simulink library "halout"  (R2021b)
settings: Solver=VariableStepAuto  StartTime=0.0  StopTime=10.0  RelTol=1e-3
undefined symbols (not defined in the file): C_TASK_5MS_S, FALSE, KHAL_CAN1FDAPS3E2E_flg, KHAL_CAN1FDAPS3TxReq_flg, KHAL_CAN1FDVCU2E2E_flg, KHAL_CAN1FDVCU2TxReq_flg, KHAL_CAN1FDVCU3E2E_flg, KHAL_CAN1FDVCU3TxReq_flg, KHAL_CAN1TxReq_flg, KHAL_CAN2TxReq_flg, KHAL_CAN3FDVCU1TxReq_flg, KHAL_CAN3FDVCU2E2E_flg, KHAL_CAN3FDVCU2TxReq_flg, KHAL_CAN3TxReq_flg, KHAL_CAN4FDVCU1E2E_flg, KHAL_CAN4FDVCU1TxReq_flg, KHAL_CAN4TxReq_flg, KHAL_CAN5TxReq_flg, ONE_INT, TRUE, ZERO_INT
libraries: FVT_lib x383, simulink x179
(part 14 of 20)

== system halout/HAL_OUT/CAN2/FD_BCM2_0x217/AmbLightBreath2 ==
  AmbLightBreath2 : Inport
  Data Type Conversion : DataTypeConversion  OutDataTypeStr=uint8  RndMeth=Round
  CAN2_AmbLightBreath2 : Outport
  wires:
  Data Type Conversion/1 -> CAN2_AmbLightBreath2/1
  AmbLightBreath2/1 -> Data Type Conversion/1

== system halout/HAL_OUT/CAN2/FD_BCM2_0x217/AmbLightBreath3 ==
  AmbLightBreath3 : Inport
  Data Type Conversion : DataTypeConversion  OutDataTypeStr=uint8  RndMeth=Round
  CAN2_AmbLightBreath3 : Outport
  wires:
  Data Type Conversion/1 -> CAN2_AmbLightBreath3/1
  AmbLightBreath3/1 -> Data Type Conversion/1

== system halout/HAL_OUT/CAN2/FD_BCM2_0x217/AmbLightBrightness1 ==
  AmbLightBrightness1 : Inport
  Data Type Conversion : DataTypeConversion  OutDataTypeStr=uint8  RndMeth=Round
  CAN2_AmbLightBrightness1 : Outport
  wires:
  Data Type Conversion/1 -> CAN2_AmbLightBrightness1/1
  AmbLightBrightness1/1 -> Data Type Conversion/1

== system halout/HAL_OUT/CAN2/FD_BCM2_0x217/AmbLightBrightness2 ==
  AmbLightBrightness2 : Inport
  Data Type Conversion : DataTypeConversion  OutDataTypeStr=uint8  RndMeth=Round
  CAN2_AmbLightBrightness2 : Outport
  wires:
  Data Type Conversion/1 -> CAN2_AmbLightBrightness2/1
  AmbLightBrightness2/1 -> Data Type Conversion/1

== system halout/HAL_OUT/CAN2/FD_BCM2_0x217/AmbLightBrightness3 ==
  AmbLightBrightness3 : Inport
  Data Type Conversion : DataTypeConversion  OutDataTypeStr=uint8  RndMeth=Round
  CAN2_AmbLightBrightness3 : Outport
  wires:
  Data Type Conversion/1 -> CAN2_AmbLightBrightness3/1
  AmbLightBrightness3/1 -> Data Type Conversion/1

== system halout/HAL_OUT/CAN2/FD_BCM2_0x217/AmbLightColor1 ==
  AmbLightColor1 : Inport
  Data Type Conversion : DataTypeConversion  OutDataTypeStr=uint8  RndMeth=Round
  CAN2_AmbLightColor1 : Outport
  wires:
  Data Type Conversion/1 -> CAN2_AmbLightColor1/1
  AmbLightColor1/1 -> Data Type Conversion/1

== system halout/HAL_OUT/CAN2/FD_BCM2_0x217/AmbLightColor2 ==
  AmbLightColor2 : Inport
  Data Type Conversion : DataTypeConversion  OutDataTypeStr=uint8  RndMeth=Round
  CAN2_AmbLightColor2 : Outport
  wires:
  Data Type Conversion/1 -> CAN2_AmbLightColor2/1
  AmbLightColor2/1 -> Data Type Conversion/1

== system halout/HAL_OUT/CAN2/FD_BCM2_0x217/AmbLightColor3 ==
  AmbLightColor3 : Inport
  Data Type Conversion : DataTypeConversion  OutDataTypeStr=uint8  RndMeth=Round
  CAN2_AmbLightColor3 : Outport
  wires:
  Data Type Conversion/1 -> CAN2_AmbLightColor3/1
  AmbLightColor3/1 -> Data Type Conversion/1

== system halout/HAL_OUT/CAN2/FD_BCM2_0x217/LampPwr ==
  LampPwr : Inport
  Data Type Conversion : DataTypeConversion  OutDataTypeStr=uint8  RndMeth=Round
  CAN2_LampPwr : Outport
  wires:
  Data Type Conversion/1 -> CAN2_LampPwr/1
  LampPwr/1 -> Data Type Conversion/1

== system halout/HAL_OUT/CAN2/FD_BCM2_0x217/User1AmbLightColor ==
  User1AmbLightColor : Inport
  Data Type Conversion : DataTypeConversion  OutDataTypeStr=uint8  RndMeth=Round
  CAN2_User1AmbLightColor : Outport
  wires:
  Data Type Conversion/1 -> CAN2_User1AmbLightColor/1
  User1AmbLightColor/1 -> Data Type Conversion/1

== system halout/HAL_OUT/CAN2/FD_BCM2_0x217/User1DrAmbLightBrightness ==
  User1DrAmbLightBrightness : Inport
  Data Type Conversion : DataTypeConversion  OutDataTypeStr=uint8  RndMeth=Round
  CAN2_User1DrAmbLightBrightness : Outport
  wires:
  Data Type Conversion/1 -> CAN2_User1DrAmbLightBrightness/1
  User1DrAmbLightBrightness/1 -> Data Type Conversion/1

== system halout/HAL_OUT/CAN2/FD_BCM2_0x217/User1IPAmbLightBrightness ==
  User1IPAmbLightBrightness : Inport
  Data Type Conversion : DataTypeConversion  OutDataTypeStr=uint8  RndMeth=Round
  CAN2_User1IPAmbLightBrightness : Outport
  wires:
  Data Type Conversion/1 -> CAN2_User1IPAmbLightBrightness/1
  User1IPAmbLightBrightness/1 -> Data Type Conversion/1

== system halout/HAL_OUT/CAN2/FD_BCM2_0x217/User2AmbLightColor ==
  User2AmbLightColor : Inport
  Data Type Conversion : DataTypeConversion  OutDataTypeStr=uint8  RndMeth=Round
  CAN2_User2AmbLightColor : Outport
  wires:
  Data Type Conversion/1 -> CAN2_User2AmbLightColor/1
  User2AmbLightColor/1 -> Data Type Conversion/1

== system halout/HAL_OUT/CAN2/FD_BCM2_0x217/User2DrAmbLightBrightness ==
  User2DrAmbLightBrightness : Inport
  Data Type Conversion : DataTypeConversion  OutDataTypeStr=uint8  RndMeth=Round
  CAN2_User2DrAmbLightBrightness : Outport
  wires:
  Data Type Conversion/1 -> CAN2_User2DrAmbLightBrightness/1
  User2DrAmbLightBrightness/1 -> Data Type Conversion/1

== system halout/HAL_OUT/CAN2/FD_BCM2_0x217/User2IPAmbLightBrightness ==
  User2IPAmbLightBrightness : Inport
  Data Type Conversion : DataTypeConversion  OutDataTypeStr=uint8  RndMeth=Round
  CAN2_User2IPAmbLightBrightness : Outport
  wires:
  Data Type Conversion/1 -> CAN2_User2IPAmbLightBrightness/1
  User2IPAmbLightBrightness/1 -> Data Type Conversion/1

== system halout/HAL_OUT/CAN2/FD_BCM2_0x217/User3AmbLightColor ==
  User3AmbLightColor : Inport
  Data Type Conversion : DataTypeConversion  OutDataTypeStr=uint8  RndMeth=Round
  CAN2_User3AmbLightColor : Outport
  wires:
  Data Type Conversion/1 -> CAN2_User3AmbLightColor/1
  User3AmbLightColor/1 -> Data Type Conversion/1

== system halout/HAL_OUT/CAN2/FD_BCM2_0x217/User3DrAmbLightBrightness ==
  User3DrAmbLightBrightness : Inport
  Data Type Conversion : DataTypeConversion  OutDataTypeStr=uint8  RndMeth=Round
  CAN2_User3DrAmbLightBrightness : Outport
  wires:
  Data Type Conversion/1 -> CAN2_User3DrAmbLightBrightness/1
  User3DrAmbLightBrightness/1 -> Data Type Conversion/1

== system halout/HAL_OUT/CAN2/FD_BCM2_0x217/User3IPAmbLightBrightness ==
  User3IPAmbLightBrightness : Inport
  Data Type Conversion : DataTypeConversion  OutDataTypeStr=uint8  RndMeth=Round
  CAN2_User3IPAmbLightBrightness : Outport
  wires:
  Data Type Conversion/1 -> CAN2_User3IPAmbLightBrightness/1
  User3IPAmbLightBrightness/1 -> Data Type Conversion/1

== system halout/HAL_OUT/CAN2/FD_BCM2_0x217/User4AmbLightColor ==
  User4AmbLightColor : Inport
  Data Type Conversion : DataTypeConversion  OutDataTypeStr=uint8  RndMeth=Round
  CAN2_User4AmbLightColor : Outport
  wires:
  Data Type Conversion/1 -> CAN2_User4AmbLightColor/1
  User4AmbLightColor/1 -> Data Type Conversion/1

== system halout/HAL_OUT/CAN2/FD_BCM2_0x217/User4DrAmbLightBrightness ==
  User4DrAmbLightBrightness : Inport
  Data Type Conversion : DataTypeConversion  OutDataTypeStr=uint8  RndMeth=Round
  CAN2_User4DrAmbLightBrightness : Outport
  wires:
  Data Type Conversion/1 -> CAN2_User4DrAmbLightBrightness/1
  User4DrAmbLightBrightness/1 -> Data Type Conversion/1

== system halout/HAL_OUT/CAN2/FD_BCM2_0x217/User4IPAmbLightBrightness ==
  User4IPAmbLightBrightness : Inport
  Data Type Conversion : DataTypeConversion  OutDataTypeStr=uint8  RndMeth=Round
  CAN2_User4IPAmbLightBrightness : Outport
  wires:
  Data Type Conversion/1 -> CAN2_User4IPAmbLightBrightness/1
  User4IPAmbLightBrightness/1 -> Data Type Conversion/1

== system halout/HAL_OUT/CAN2/FD_BCM2_0x217/User5AmbLightColor ==
  User5AmbLightColor : Inport
  Data Type Conversion : DataTypeConversion  OutDataTypeStr=uint8  RndMeth=Round
  CAN2_User5AmbLightColor : Outport
  wires:
  Data Type Conversion/1 -> CAN2_User5AmbLightColor/1
  User5AmbLightColor/1 -> Data Type Conversion/1

== system halout/HAL_OUT/CAN2/FD_BCM2_0x217/User5DrAmbLightBrightness ==
  User5DrAmbLightBrightness : Inport
  Data Type Conversion : DataTypeConversion  OutDataTypeStr=uint8  RndMeth=Round
  CAN2_User5DrAmbLightBrightness : Outport
  wires:
  Data Type Conversion/1 -> CAN2_User5DrAmbLightBrightness/1
  User5DrAmbLightBrightness/1 -> Data Type Conversion/1

== system halout/HAL_OUT/CAN2/FD_BCM2_0x217/User5IPAmbLightBrightness ==
  User5IPAmbLightBrightness : Inport
  Data Type Conversion : DataTypeConversion  OutDataTypeStr=uint8  RndMeth=Round
  CAN2_User5IPAmbLightBrightness : Outport
  wires:
  Data Type Conversion/1 -> CAN2_User5IPAmbLightBrightness/1
  User5IPAmbLightBrightness/1 -> Data Type Conversion/1

== system halout/HAL_OUT/CAN2/FD_BCM2_0x217/User6AmbLightColor ==
  User6AmbLightColor : Inport
  Data Type Conversion : DataTypeConversion  OutDataTypeStr=uint8  RndMeth=Round
  CAN2_User6AmbLightColor : Outport
  wires:
  Data Type Conversion/1 -> CAN2_User6AmbLightColor/1
  User6AmbLightColor/1 -> Data Type Conversion/1

== system halout/HAL_OUT/CAN2/FD_BCM2_0x217/User6DrAmbLightBrightness ==
  User6DrAmbLightBrightness : Inport
  Data Type Conversion : DataTypeConversion  OutDataTypeStr=uint8  RndMeth=Round
  CAN2_User6DrAmbLightBrightness : Outport
  wires:
  Data Type Conversion/1 -> CAN2_User6DrAmbLightBrightness/1
  User6DrAmbLightBrightness/1 -> Data Type Conversion/1

== system halout/HAL_OUT/CAN2/FD_BCM2_0x217/User6IPAmbLightBrightness ==
  User6IPAmbLightBrightness : Inport
  Data Type Conversion : DataTypeConversion  OutDataTypeStr=uint8  RndMeth=Round
  CAN2_User6IPAmbLightBrightness : Outport
  wires:
  Data Type Conversion/1 -> CAN2_User6IPAmbLightBrightness/1
  User6IPAmbLightBrightness/1 -> Data Type Conversion/1

== system halout/HAL_OUT/CAN2/FD_THCM1_0x182/BatteryMode ==
  BatteryMode : Inport
  Data Type Conversion : DataTypeConversion  OutDataTypeStr=uint8  RndMeth=Round
  CAN2_BatteryMode : Outport
  wires:
  Data Type Conversion/1 -> CAN2_BatteryMode/1
  BatteryMode/1 -> Data Type Conversion/1

== system halout/HAL_OUT/CAN2/FD_THCM1_0x182/CCUACLampSts ==
  CCUACLampSts : Inport
  Data Type Conversion : DataTypeConversion  OutDataTypeStr=uint8  RndMeth=Round
  CAN2_CCU_ACLampSts : Outport
  wires:
  Data Type Conversion/1 -> CAN2_CCU_ACLampSts/1
  CCUACLampSts/1 -> Data Type Conversion/1

== system halout/HAL_OUT/CAN2/FD_THCM1_0x182/CCUACMaxLampSts ==
  CCUACMaxLampSts : Inport
  Data Type Conversion : DataTypeConversion  OutDataTypeStr=uint8  RndMeth=Round
  CAN2_CCU_ACMaxLampSts : Outport
  wires:
  Data Type Conversion/1 -> CAN2_CCU_ACMaxLampSts/1
  CCUACMaxLampSts/1 -> Data Type Conversion/1

== system halout/HAL_OUT/CAN2/FD_THCM1_0x182/CCUAutoLampSts ==
  CCUAutoLampSts : Inport
  Data Type Conversion : DataTypeConversion  OutDataTypeStr=uint8  RndMeth=Round
  CAN2_CCU_AutoLampSts : Outport
  wires:
  Data Type Conversion/1 -> CAN2_CCU_AutoLampSts/1
  CCUAutoLampSts/1 -> Data Type Conversion/1

== system halout/HAL_OUT/CAN2/FD_THCM1_0x182/CCUAutoMidLampSts ==
  CCUAutoMidLampSts : Inport
  Data Type Conversion : DataTypeConversion  OutDataTypeStr=uint8  RndMeth=Round
  CAN2_CCU_AutoMidLampSts : Outport
  wires:
  Data Type Conversion/1 -> CAN2_CCU_AutoMidLampSts/1
  CCUAutoMidLampSts/1 -> Data Type Conversion/1

== system halout/HAL_OUT/CAN2/FD_THCM1_0x182/CCUDispalyRequest ==
  CCUDispalyRequest : Inport
  Data Type Conversion : DataTypeConversion  OutDataTypeStr=uint8  RndMeth=Round
  CAN2_CCU_Dispaly_Request : Outport
  wires:
  Data Type Conversion/1 -> CAN2_CCU_Dispaly_Request/1
  CCUDispalyRequest/1 -> Data Type Conversion/1

== system halout/HAL_OUT/CAN2/FD_THCM1_0x182/CCUEcoSts ==
  CCUEcoSts : Inport
  Data Type Conversion : DataTypeConversion  OutDataTypeStr=uint8  RndMeth=Round
  CAN2_CCU_EcoSts : Outport
  wires:
  Data Type Conversion/1 -> CAN2_CCU_EcoSts/1
  CCUEcoSts/1 -> Data Type Conversion/1

== system halout/HAL_OUT/CAN2/FD_THCM1_0x182/CCUFrtOnOffLampSts ==
  CCUFrtOnOffLampSts : Inport
  Data Type Conversion : DataTypeConversion  OutDataTypeStr=uint8  RndMeth=Round
  CAN2_CCU_FrtOnOffLampSts : Outport
  wires:
  Data Type Conversion/1 -> CAN2_CCU_FrtOnOffLampSts/1
  CCUFrtOnOffLampSts/1 -> Data Type Conversion/1

== system halout/HAL_OUT/CAN2/FD_THCM1_0x182/CCUHEATMaxLampSts ==
  CCUHEATMaxLampSts : Inport
  Data Type Conversion : DataTypeConversion  OutDataTypeStr=uint8  RndMeth=Round
  CAN2_CCU_HEATMaxLampSts : Outport
  wires:
  Data Type Conversion/1 -> CAN2_CCU_HEATMaxLampSts/1
  CCUHEATMaxLampSts/1 -> Data Type Conversion/1

== system halout/HAL_OUT/CAN2/FD_THCM1_0x182/CCURrOnOffLampSts ==
  CCURrOnOffLampSts : Inport
  Data Type Conversion : DataTypeConversion  OutDataTypeStr=uint8  RndMeth=Round
  CAN2_CCU_RrOnOffLampSts : Outport
  wires:
  Data Type Conversion/1 -> CAN2_CCU_RrOnOffLampSts/1
  CCURrOnOffLampSts/1 -> Data Type Conversion/1

== system halout/HAL_OUT/CAN2/FD_THCM1_0x182/CCUSyncLampSts ==
  CCUSyncLampSts : Inport
  Data Type Conversion : DataTypeConversion  OutDataTypeStr=uint8  RndMeth=Round
  CAN2_CCU_SyncLampSts : Outport
  wires:
  Data Type Conversion/1 -> CAN2_CCU_SyncLampSts/1
  CCUSyncLampSts/1 -> Data Type Conversion/1

== system halout/HAL_OUT/CAN2/FD_THCM1_0x182/CabinMode ==
  CabinMode : Inport
  Data Type Conversion : DataTypeConversion  OutDataTypeStr=uint8  RndMeth=Round
  CAN2_CabinMode : Outport
  wires:
  Data Type Conversion/1 -> CAN2_CabinMode/1
  CabinMode/1 -> Data Type Conversion/1

== system halout/HAL_OUT/CAN2/FD_THCM1_0x182/EDriveMode ==
  EDriveMode : Inport
  Data Type Conversion : DataTypeConversion  OutDataTypeStr=uint8  RndMeth=Round
  CAN2_EDriveMode : Outport
  wires:
  Data Type Conversion/1 -> CAN2_EDriveMode/1
  EDriveMode/1 -> Data Type Conversion/1

== system halout/HAL_OUT/CAN2/FD_THCM1_0x182/FDAGSCmd ==
  FDAGSCmd : Inport
  Data Type Conversion : DataTypeConversion  OutDataTypeStr=uint8  RndMeth=Round
  CAN2_FD_AGS_Cmd : Outport
  wires:
  Data Type Conversion/1 -> CAN2_FD_AGS_Cmd/1
  FDAGSCmd/1 -> Data Type Conversion/1

== system halout/HAL_OUT/CAN2/FD_THCM1_0x182/FDRecyAutoCmd ==
  FDRecyAutoCmd : Inport
  Data Type Conversion : DataTypeConversion  OutDataTypeStr=uint8  RndMeth=Round
  CAN2_FD_RecyAuto_Cmd : Outport
  wires:
  Data Type Conversion/1 -> CAN2_FD_RecyAuto_Cmd/1
  FDRecyAutoCmd/1 -> Data Type Conversion/1

== system halout/HAL_OUT/CAN2/FD_THCM1_0x182/FrCoolantflow ==
  FrCoolantflow : Inport
  Data Type Conversion : DataTypeConversion  OutDataTypeStr=uint8  RndMeth=Round
  convert_out : FVT_lib/hal/convert_out  gain=0.25  offset=0
  CAN2_Fr_Coolantflow : Outport
  wires:
  Data Type Conversion/1 -> CAN2_Fr_Coolantflow/1
  convert_out/1 -> Data Type Conversion/1
  FrCoolantflow/1 -> convert_out/1

== system halout/HAL_OUT/CAN2/FD_THCM1_0x182/FrCoolanttemp ==
  FrCoolanttemp : Inport
  Data Type Conversion : DataTypeConversion  OutDataTypeStr=uint16  RndMeth=Round
  convert_out : FVT_lib/hal/convert_out  gain=1  offset=-40
  CAN2_Fr_Coolanttemp : Outport
  wires:
  Data Type Conversion/1 -> CAN2_Fr_Coolanttemp/1
  convert_out/1 -> Data Type Conversion/1
  FrCoolanttemp/1 -> convert_out/1

== system halout/HAL_OUT/CAN2/FD_THCM1_0x182/HPThermalRecoveryReq ==
  HPThermalRecoveryReq : Inport
  Data Type Conversion : DataTypeConversion  OutDataTypeStr=uint8  RndMeth=Round
  CAN2_HPThermalRecoveryReq : Outport
  wires:
  Data Type Conversion/1 -> CAN2_HPThermalRecoveryReq/1
  HPThermalRecoveryReq/1 -> Data Type Conversion/1

== system halout/HAL_OUT/CAN2/FD_THCM1_0x182/RrCoolantflow ==
  RrCoolantflow : Inport
  Data Type Conversion : DataTypeConversion  OutDataTypeStr=uint8  RndMeth=Round
  convert_out : FVT_lib/hal/convert_out  gain=0.25  offset=0
  CAN2_Rr_Coolantflow : Outport
  wires:
  Data Type Conversion/1 -> CAN2_Rr_Coolantflow/1
  convert_out/1 -> Data Type Conversion/1
  RrCoolantflow/1 -> convert_out/1

== system halout/HAL_OUT/CAN2/FD_THCM1_0x182/RrCoolanttemp ==
  RrCoolanttemp : Inport
  Data Type Conversion : DataTypeConversion  OutDataTypeStr=uint16  RndMeth=Round
  convert_out : FVT_lib/hal/convert_out  gain=1  offset=-40
  CAN2_Rr_Coolanttemp : Outport
  wires:
  Data Type Conversion/1 -> CAN2_Rr_Coolanttemp/1
  convert_out/1 -> Data Type Conversion/1
  RrCoolanttemp/1 -> convert_out/1

== system halout/HAL_OUT/CAN2/FD_THCM1_0x182/sigAirIntenZon1St ==
  sigAirIntenZon1St : Inport
  Data Type Conversion : DataTypeConversion  OutDataTypeStr=uint8  RndMeth=Round
  CAN2_sigAirIntenZon1St : Outport
  wires:
  Data Type Conversion/1 -> CAN2_sigAirIntenZon1St/1
  sigAirIntenZon1St/1 -> Data Type Conversion/1

== system halout/HAL_OUT/CAN2/FD_THCM1_0x182/sigAirIntenZon3St ==
  sigAirIntenZon3St : Inport
  Data Type Conversion : DataTypeConversion  OutDataTypeStr=uint8  RndMeth=Round
  CAN2_sigAirIntenZon3St : Outport
  wires:
  Data Type Conversion/1 -> CAN2_sigAirIntenZon3St/1
  sigAirIntenZon3St/1 -> Data Type Conversion/1

== system halout/HAL_OUT/CAN2/FD_THCM1_0x182/sigAmbAirT ==
  sigAmbAirT : Inport
  Data Type Conversion : DataTypeConversion  OutDataTypeStr=uint8  RndMeth=Round
  convert_out : FVT_lib/hal/convert_out  gain=0.5  offset=-40
  CAN2_sigAmbAirT : Outport
  wires:
  Data Type Conversion/1 -> CAN2_sigAmbAirT/1
  convert_out/1 -> Data Type Conversion/1
  sigAmbAirT/1 -> convert_out/1

== system halout/HAL_OUT/CAN2/FD_THCM1_0x182/sigCbnAirT ==
  sigCbnAirT : Inport
  Data Type Conversion : DataTypeConversion  OutDataTypeStr=uint8  RndMeth=Round
  convert_out : FVT_lib/hal/convert_out  gain=0.5  offset=-40
  CAN2_sigCbnAirT : Outport
  wires:
  Data Type Conversion/1 -> CAN2_sigCbnAirT/1
  convert_out/1 -> Data Type Conversion/1
  sigCbnAirT/1 -> convert_out/1

== system halout/HAL_OUT/CAN2/FD_THCM1_0x182/sigCbnPTCPwrAct ==
  sigCbnPTCPwrAct : Inport
  Data Type Conversion : DataTypeConversion  OutDataTypeStr=uint8  RndMeth=Round
  convert_out : FVT_lib/hal/convert_out  gain=50  offset=0
  CAN2_sigCbnPTCPwrAct : Outport
  wires:
  Data Type Conversion/1 -> CAN2_sigCbnPTCPwrAct/1
  convert_out/1 -> Data Type Conversion/1
  sigCbnPTCPwrAct/1 -> convert_out/1

== system halout/HAL_OUT/CAN2/FD_THCM1_0x182/sigCbnSolarLeft ==
  sigCbnSolarLeft : Inport
  Data Type Conversion : DataTypeConversion  OutDataTypeStr=uint8  RndMeth=Round
  convert_out : FVT_lib/hal/convert_out  gain=5  offset=0
  CAN2_sigCbnSolarLeft : Outport
  wires:
  Data Type Conversion/1 -> CAN2_sigCbnSolarLeft/1
  convert_out/1 -> Data Type Conversion/1
  sigCbnSolarLeft/1 -> convert_out/1

== system halout/HAL_OUT/CAN2/FD_THCM1_0x182/sigCbnSolarRight ==
  sigCbnSolarRight : Inport
  Data Type Conversion : DataTypeConversion  OutDataTypeStr=uint8  RndMeth=Round
  convert_out : FVT_lib/hal/convert_out  gain=5  offset=0
  CAN2_sigCbnSolarRight : Outport
  wires:
  Data Type Conversion/1 -> CAN2_sigCbnSolarRight/1
  convert_out/1 -> Data Type Conversion/1
  sigCbnSolarRight/1 -> convert_out/1

== system halout/HAL_OUT/CAN2/FD_THCM1_0x182/sigClmtCmprPwrAct ==
  sigClmtCmprPwrAct : Inport
  Data Type Conversion : DataTypeConversion  OutDataTypeStr=uint8  RndMeth=Round
  convert_out : FVT_lib/hal/convert_out  gain=50  offset=0
  CAN2_sigClmtCmprPwrAct : Outport
  wires:
  Data Type Conversion/1 -> CAN2_sigClmtCmprPwrAct/1
  convert_out/1 -> Data Type Conversion/1
  sigClmtCmprPwrAct/1 -> convert_out/1

== system halout/HAL_OUT/CAN2/FD_THCM1_0x182/sigClntTHvBattOut ==
  sigClntTHvBattOut : Inport
  Data Type Conversion : DataTypeConversion  OutDataTypeStr=uint8  RndMeth=Round
  convert_out : FVT_lib/hal/convert_out  gain=0.5  offset=-40
  CAN2_sigClntTHvBattOut : Outport
  wires:
  Data Type Conversion/1 -> CAN2_sigClntTHvBattOut/1
  convert_out/1 -> Data Type Conversion/1
  sigClntTHvBattOut/1 -> convert_out/1

== system halout/HAL_OUT/CAN2/FD_THCM1_0x182/sigDfrstSt ==
  sigDfrstSt : Inport
  Data Type Conversion : DataTypeConversion  OutDataTypeStr=uint8  RndMeth=Round
  CAN2_sigDfrstSt : Outport
  wires:
  Data Type Conversion/1 -> CAN2_sigDfrstSt/1
  sigDfrstSt/1 -> Data Type Conversion/1

== system halout/HAL_OUT/CAN2/FD_THCM1_0x182/sigHvacSt ==
  sigHvacSt : Inport
  Data Type Conversion : DataTypeConversion  OutDataTypeStr=uint8  RndMeth=Round
  CAN2_sigHvacSt : Outport
  wires:
  Data Type Conversion/1 -> CAN2_sigHvacSt/1
  sigHvacSt/1 -> Data Type Conversion/1

== system halout/HAL_OUT/CAN2/FD_THCM1_0x182/sigRecircSt ==
  sigRecircSt : Inport
  Data Type Conversion : DataTypeConversion  OutDataTypeStr=uint8  RndMeth=Round
  CAN2_sigRecircSt : Outport
  wires:
  Data Type Conversion/1 -> CAN2_sigRecircSt/1
  sigRecircSt/1 -> Data Type Conversion/1

== system halout/HAL_OUT/CAN2/FD_THCM1_0x182/sigSetTempZon1St ==
  sigSetTempZon1St : Inport
  Data Type Conversion : DataTypeConversion  OutDataTypeStr=uint8  RndMeth=Round
  convert_out : FVT_lib/hal/convert_out  gain=0.5  offset=17
  CAN2_sigSetTempZon1St : Outport
  wires:
  Data Type Conversion/1 -> CAN2_sigSetTempZon1St/1
  convert_out/1 -> Data Type Conversion/1
  sigSetTempZon1St/1 -> convert_out/1

== system halout/HAL_OUT/CAN2/FD_THCM1_0x182/sigSetTempZon2St ==
  sigSetTempZon2St : Inport
  Data Type Conversion : DataTypeConversion  OutDataTypeStr=uint8  RndMeth=Round
  convert_out : FVT_lib/hal/convert_out  gain=0.5  offset=17
  CAN2_sigSetTempZon2St : Outport
  wires:
  Data Type Conversion/1 -> CAN2_sigSetTempZon2St/1
  convert_out/1 -> Data Type Conversion/1
  sigSetTempZon2St/1 -> convert_out/1

== system halout/HAL_OUT/CAN2/FD_THCM1_0x182/sigSetTempZon3St ==
  sigSetTempZon3St : Inport
  Data Type Conversion : DataTypeConversion  OutDataTypeStr=uint8  RndMeth=Round
  convert_out : FVT_lib/hal/convert_out  gain=0.5  offset=17
  CAN2_sigSetTempZon3St : Outport
  wires:
  Data Type Conversion/1 -> CAN2_sigSetTempZon3St/1
  convert_out/1 -> Data Type Conversion/1
  sigSetTempZon3St/1 -> convert_out/1

== system halout/HAL_OUT/CAN2/FD_THCM1_0x182/sigWindDirZon1St ==
  sigWindDirZon1St : Inport
  Data Type Conversion : DataTypeConversion  OutDataTypeStr=uint8  RndMeth=Round
  CAN2_sigWindDirZon1St : Outport
  wires:
  Data Type Conversion/1 -> CAN2_sigWindDirZon1St/1
  sigWindDirZon1St/1 -> Data Type Conversion/1

== system halout/HAL_OUT/CAN2/FD_THCM1_0x182/sigWindDirZon3St ==
  sigWindDirZon3St : Inport
  Data Type Conversion : DataTypeConversion  OutDataTypeStr=uint8  RndMeth=Round
  CAN2_sigWindDirZon3St : Outport
  wires:
  Data Type Conversion/1 -> CAN2_sigWindDirZon3St/1
  sigWindDirZon3St/1 -> Data Type Conversion/1

== system halout/HAL_OUT/CAN2/FD_TPMS1_0x435/AutoLTips ==
  AutoLTips : Inport
  Data Type Conversion : DataTypeConversion  OutDataTypeStr=uint8  RndMeth=Round
  CAN2_AutoLTips : Outport
  wires:
  Data Type Conversion/1 -> CAN2_AutoLTips/1
  AutoLTips/1 -> Data Type Conversion/1

== system halout/HAL_OUT/CAN2/FD_TPMS1_0x435/CWheelTips ==
  CWheelTips : Inport
  Data Type Conversion : DataTypeConversion  OutDataTypeStr=uint8  RndMeth=Round
  CAN2_CWheelTips : Outport
  wires:
  Data Type Conversion/1 -> CAN2_CWheelTips/1
  CWheelTips/1 -> Data Type Conversion/1

== system halout/HAL_OUT/CAN2/FD_TPMS1_0x435/LFBatWarn ==
  LFBatWarn : Inport
  Data Type Conversion : DataTypeConversion  OutDataTypeStr=uint8  RndMeth=Round
  CAN2_LFBatWarn : Outport
  wires:
  Data Type Conversion/1 -> CAN2_LFBatWarn/1
  LFBatWarn/1 -> Data Type Conversion/1

== system halout/HAL_OUT/CAN2/FD_TPMS1_0x435/LFPressIndi ==
  LFPressIndi : Inport
  Data Type Conversion : DataTypeConversion  OutDataTypeStr=uint8  RndMeth=Round
  CAN2_LFPressIndi : Outport
  wires:
  Data Type Conversion/1 -> CAN2_LFPressIndi/1
  LFPressIndi/1 -> Data Type Conversion/1

== system halout/HAL_OUT/CAN2/FD_TPMS1_0x435/LFSensorFail ==
  LFSensorFail : Inport
  Data Type Conversion : DataTypeConversion  OutDataTypeStr=uint8  RndMeth=Round
  CAN2_LFSensorFail : Outport
  wires:
  Data Type Conversion/1 -> CAN2_LFSensorFail/1
  LFSensorFail/1 -> Data Type Conversion/1

== system halout/HAL_OUT/CAN2/FD_TPMS1_0x435/LFSensorMode ==
  LFSensorMode : Inport
  Data Type Conversion : DataTypeConversion  OutDataTypeStr=uint8  RndMeth=Round
  CAN2_LFSensorMode : Outport
  wires:
  Data Type Conversion/1 -> CAN2_LFSensorMode/1
  LFSensorMode/1 -> Data Type Conversion/1

== system halout/HAL_OUT/CAN2/FD_TPMS1_0x435/LFWheelDebug ==
  LFWheelDebug : Inport
  Data Type Conversion : DataTypeConversion  OutDataTypeStr=uint8  RndMeth=Round
  CAN2_LFWheelDebug : Outport
  wires:
  Data Type Conversion/1 -> CAN2_LFWheelDebug/1
  LFWheelDebug/1 -> Data Type Conversion/1

== system halout/HAL_OUT/CAN2/FD_TPMS1_0x435/LFWheelPSW ==
  LFWheelPSW : Inport
  Data Type Conversion : DataTypeConversion  OutDataTypeStr=uint8  RndMeth=Round
  CAN2_LFWheelPSW : Outport
  wires:
  Data Type Conversion/1 -> CAN2_LFWheelPSW/1
  LFWheelPSW/1 -> Data Type Conversion/1

== system halout/HAL_OUT/CAN2/FD_TPMS1_0x435/LFWheelPress ==
  LFWheelPress : Inport
  Data Type Conversion : DataTypeConversion  OutDataTypeStr=uint8  RndMeth=Round
  CAN2_LFWheelPress : Outport
  wires:
  Data Type Conversion/1 -> CAN2_LFWheelPress/1
  LFWheelPress/1 -> Data Type Conversion/1

== system halout/HAL_OUT/CAN2/FD_TPMS1_0x435/LFWheelTemp ==
  LFWheelTemp : Inport
  Data Type Conversion : DataTypeConversion  OutDataTypeStr=uint8  RndMeth=Round
  convert_out : FVT_lib/hal/convert_out  gain=1  offset=-40
  CAN2_LFWheelTemp : Outport
  wires:
  Data Type Conversion/1 -> CAN2_LFWheelTemp/1
  convert_out/1 -> Data Type Conversion/1
  LFWheelTemp/1 -> convert_out/1

== system halout/HAL_OUT/CAN2/FD_TPMS1_0x435/LFWheelTmpIndi ==
  LFWheelTmpIndi : Inport
  Data Type Conversion : DataTypeConversion  OutDataTypeStr=uint8  RndMeth=Round
  CAN2_LFWheelTmpIndi : Outport
  wires:
  Data Type Conversion/1 -> CAN2_LFWheelTmpIndi/1
  LFWheelTmpIndi/1 -> Data Type Conversion/1

== system halout/HAL_OUT/CAN2/FD_TPMS1_0x435/LRBatWarn ==
  LRBatWarn : Inport
  Data Type Conversion : DataTypeConversion  OutDataTypeStr=uint8  RndMeth=Round
  CAN2_LRBatWarn : Outport
  wires:
  Data Type Conversion/1 -> CAN2_LRBatWarn/1
  LRBatWarn/1 -> Data Type Conversion/1

== system halout/HAL_OUT/CAN2/FD_TPMS1_0x435/LRPressIndi ==
  LRPressIndi : Inport
  Data Type Conversion : DataTypeConversion  OutDataTypeStr=uint8  RndMeth=Round
  CAN2_LRPressIndi : Outport
  wires:
  Data Type Conversion/1 -> CAN2_LRPressIndi/1
  LRPressIndi/1 -> Data Type Conversion/1

== system halout/HAL_OUT/CAN2/FD_TPMS1_0x435/LRSensorFail ==
  LRSensorFail : Inport
  Data Type Conversion : DataTypeConversion  OutDataTypeStr=uint8  RndMeth=Round
  CAN2_LRSensorFail : Outport
  wires:
  Data Type Conversion/1 -> CAN2_LRSensorFail/1
  LRSensorFail/1 -> Data Type Conversion/1

== system halout/HAL_OUT/CAN2/FD_TPMS1_0x435/LRSensorMode ==
  LRSensorMode : Inport
  Data Type Conversion : DataTypeConversion  OutDataTypeStr=uint8  RndMeth=Round
  CAN2_LRSensorMode : Outport
  wires:
  Data Type Conversion/1 -> CAN2_LRSensorMode/1
  LRSensorMode/1 -> Data Type Conversion/1

== system halout/HAL_OUT/CAN2/FD_TPMS1_0x435/LRWheelDebug ==
  LRWheelDebug : Inport
  Data Type Conversion : DataTypeConversion  OutDataTypeStr=uint8  RndMeth=Round
  CAN2_LRWheelDebug : Outport
  wires:
  Data Type Conversion/1 -> CAN2_LRWheelDebug/1
  LRWheelDebug/1 -> Data Type Conversion/1

== system halout/HAL_OUT/CAN2/FD_TPMS1_0x435/LRWheelPSW ==
  LRWheelPSW : Inport
  Data Type Conversion : DataTypeConversion  OutDataTypeStr=uint8  RndMeth=Round
  CAN2_LRWheelPSW : Outport
  wires:
  Data Type Conversion/1 -> CAN2_LRWheelPSW/1
  LRWheelPSW/1 -> Data Type Conversion/1

== system halout/HAL_OUT/CAN2/FD_TPMS1_0x435/LRWheelPress ==
  LRWheelPress : Inport
  Data Type Conversion : DataTypeConversion  OutDataTypeStr=uint8  RndMeth=Round
  CAN2_LRWheelPress : Outport
  wires:
  Data Type Conversion/1 -> CAN2_LRWheelPress/1
  LRWheelPress/1 -> Data Type Conversion/1

== system halout/HAL_OUT/CAN2/FD_TPMS1_0x435/LRWheelTemp ==
  LRWheelTemp : Inport
  Data Type Conversion : DataTypeConversion  OutDataTypeStr=uint8  RndMeth=Round
  convert_out : FVT_lib/hal/convert_out  gain=1  offset=-40
  CAN2_LRWheelTemp : Outport
  wires:
  Data Type Conversion/1 -> CAN2_LRWheelTemp/1
  convert_out/1 -> Data Type Conversion/1
  LRWheelTemp/1 -> convert_out/1

== system halout/HAL_OUT/CAN2/FD_TPMS1_0x435/LRWheelTmpIndi ==
  LRWheelTmpIndi : Inport
  Data Type Conversion : DataTypeConversion  OutDataTypeStr=uint8  RndMeth=Round
  CAN2_LRWheelTmpIndi : Outport
  wires:
  Data Type Conversion/1 -> CAN2_LRWheelTmpIndi/1
  LRWheelTmpIndi/1 -> Data Type Conversion/1

== system halout/HAL_OUT/CAN2/FD_TPMS1_0x435/RFBatWarn ==
  RFBatWarn : Inport
  Data Type Conversion : DataTypeConversion  OutDataTypeStr=uint8  RndMeth=Round
  CAN2_RFBatWarn : Outport
  wires:
  Data Type Conversion/1 -> CAN2_RFBatWarn/1
  RFBatWarn/1 -> Data Type Conversion/1

== system halout/HAL_OUT/CAN2/FD_TPMS1_0x435/RFPressIndi ==
  RFPressIndi : Inport
  Data Type Conversion : DataTypeConversion  OutDataTypeStr=uint8  RndMeth=Round
  CAN2_RFPressIndi : Outport
  wires:
  Data Type Conversion/1 -> CAN2_RFPressIndi/1
  RFPressIndi/1 -> Data Type Conversion/1

== system halout/HAL_OUT/CAN2/FD_TPMS1_0x435/RFSensorFail ==
  RFSensorFail : Inport
  Data Type Conversion : DataTypeConversion  OutDataTypeStr=uint8  RndMeth=Round
  CAN2_RFSensorFail : Outport
  wires:
  Data Type Conversion/1 -> CAN2_RFSensorFail/1
  RFSensorFail/1 -> Data Type Conversion/1

== system halout/HAL_OUT/CAN2/FD_TPMS1_0x435/RFSensorMode ==
  RFSensorMode : Inport
  Data Type Conversion : DataTypeConversion  OutDataTypeStr=uint8  RndMeth=Round
  CAN2_RFSensorMode : Outport
  wires:
  Data Type Conversion/1 -> CAN2_RFSensorMode/1
  RFSensorMode/1 -> Data Type Conversion/1

== system halout/HAL_OUT/CAN2/FD_TPMS1_0x435/RFWheelDebug ==
  RFWheelDebug : Inport
  Data Type Conversion : DataTypeConversion  OutDataTypeStr=uint8  RndMeth=Round
  CAN2_RFWheelDebug : Outport
  wires:
  Data Type Conversion/1 -> CAN2_RFWheelDebug/1
  RFWheelDebug/1 -> Data Type Conversion/1

== system halout/HAL_OUT/CAN2/FD_TPMS1_0x435/RFWheelPSW ==
  RFWheelPSW : Inport
  Data Type Conversion : DataTypeConversion  OutDataTypeStr=uint8  RndMeth=Round
  CAN2_RFWheelPSW : Outport
  wires:
  Data Type Conversion/1 -> CAN2_RFWheelPSW/1
  RFWheelPSW/1 -> Data Type Conversion/1

== system halout/HAL_OUT/CAN2/FD_TPMS1_0x435/RFWheelPress ==
  RFWheelPress : Inport
  Data Type Conversion : DataTypeConversion  OutDataTypeStr=uint8  RndMeth=Round
  CAN2_RFWheelPress : Outport
  wires:
  Data Type Conversion/1 -> CAN2_RFWheelPress/1
  RFWheelPress/1 -> Data Type Conversion/1

== system halout/HAL_OUT/CAN2/FD_TPMS1_0x435/RFWheelTemp ==
  RFWheelTemp : Inport
  Data Type Conversion : DataTypeConversion  OutDataTypeStr=uint8  RndMeth=Round
  convert_out : FVT_lib/hal/convert_out  gain=1  offset=-40
  CAN2_RFWheelTemp : Outport
  wires:
  Data Type Conversion/1 -> CAN2_RFWheelTemp/1
  convert_out/1 -> Data Type Conversion/1
  RFWheelTemp/1 -> convert_out/1

== system halout/HAL_OUT/CAN2/FD_TPMS1_0x435/RFWheelTmpIndi ==
  RFWheelTmpIndi : Inport
  Data Type Conversion : DataTypeConversion  OutDataTypeStr=uint8  RndMeth=Round
  CAN2_RFWheelTmpIndi : Outport
  wires:
  Data Type Conversion/1 -> CAN2_RFWheelTmpIndi/1
  RFWheelTmpIndi/1 -> Data Type Conversion/1

== system halout/HAL_OUT/CAN2/FD_TPMS1_0x435/RRBatWarn ==
  RRBatWarn : Inport
  Data Type Conversion : DataTypeConversion  OutDataTypeStr=uint8  RndMeth=Round
  CAN2_RRBatWarn : Outport
  wires:
  Data Type Conversion/1 -> CAN2_RRBatWarn/1
  RRBatWarn/1 -> Data Type Conversion/1

== system halout/HAL_OUT/CAN2/FD_TPMS1_0x435/RRPressIndi ==
  RRPressIndi : Inport
  Data Type Conversion : DataTypeConversion  OutDataTypeStr=uint8  RndMeth=Round
  CAN2_RRPressIndi : Outport
  wires:
  Data Type Conversion/1 -> CAN2_RRPressIndi/1
  RRPressIndi/1 -> Data Type Conversion/1

== system halout/HAL_OUT/CAN2/FD_TPMS1_0x435/RRSensorFail ==
  RRSensorFail : Inport
  Data Type Conversion : DataTypeConversion  OutDataTypeStr=uint8  RndMeth=Round
  CAN2_RRSensorFail : Outport
  wires:
  Data Type Conversion/1 -> CAN2_RRSensorFail/1
  RRSensorFail/1 -> Data Type Conversion/1

== system halout/HAL_OUT/CAN2/FD_TPMS1_0x435/RRSensorMode ==
  RRSensorMode : Inport
  Data Type Conversion : DataTypeConversion  OutDataTypeStr=uint8  RndMeth=Round
  CAN2_RRSensorMode : Outport
  wires:
  Data Type Conversion/1 -> CAN2_RRSensorMode/1
  RRSensorMode/1 -> Data Type Conversion/1

== system halout/HAL_OUT/CAN2/FD_TPMS1_0x435/RRWheelDebug ==
  RRWheelDebug : Inport
  Data Type Conversion : DataTypeConversion  OutDataTypeStr=uint8  RndMeth=Round
  CAN2_RRWheelDebug : Outport
  wires:
  Data Type Conversion/1 -> CAN2_RRWheelDebug/1
  RRWheelDebug/1 -> Data Type Conversion/1

== system halout/HAL_OUT/CAN2/FD_TPMS1_0x435/RRWheelPSW ==
  RRWheelPSW : Inport
  Data Type Conversion : DataTypeConversion  OutDataTypeStr=uint8  RndMeth=Round
  CAN2_RRWheelPSW : Outport
  wires:
  Data Type Conversion/1 -> CAN2_RRWheelPSW/1
  RRWheelPSW/1 -> Data Type Conversion/1

== system halout/HAL_OUT/CAN2/FD_TPMS1_0x435/RRWheelPress ==
  RRWheelPress : Inport
  Data Type Conversion : DataTypeConversion  OutDataTypeStr=uint8  RndMeth=Round
  CAN2_RRWheelPress : Outport
  wires:
  Data Type Conversion/1 -> CAN2_RRWheelPress/1
  RRWheelPress/1 -> Data Type Conversion/1

== system halout/HAL_OUT/CAN2/FD_TPMS1_0x435/RRWheelTemp ==
  RRWheelTemp : Inport
  Data Type Conversion : DataTypeConversion  OutDataTypeStr=uint8  RndMeth=Round
  convert_out : FVT_lib/hal/convert_out  gain=1  offset=-40
  CAN2_RRWheelTemp : Outport
  wires:
  Data Type Conversion/1 -> CAN2_RRWheelTemp/1
  convert_out/1 -> Data Type Conversion/1
  RRWheelTemp/1 -> convert_out/1

== system halout/HAL_OUT/CAN2/FD_TPMS1_0x435/RRWheelTmpIndi ==
  RRWheelTmpIndi : Inport
  Data Type Conversion : DataTypeConversion  OutDataTypeStr=uint8  RndMeth=Round
  CAN2_RRWheelTmpIndi : Outport
  wires:
  Data Type Conversion/1 -> CAN2_RRWheelTmpIndi/1
  RRWheelTmpIndi/1 -> Data Type Conversion/1

== system halout/HAL_OUT/CAN2/FD_TPMS1_0x435/TPMSCaliButtAllow ==
  TPMSCaliButtAllow : Inport
  Data Type Conversion : DataTypeConversion  OutDataTypeStr=uint8  RndMeth=Round
  CAN2_TPMS_Cali_Butt_Allow : Outport
  wires:
  Data Type Conversion/1 -> CAN2_TPMS_Cali_Butt_Allow/1
  TPMSCaliButtAllow/1 -> Data Type Conversion/1

== system halout/HAL_OUT/CAN2/FD_TPMS1_0x435/TPMSResButtAllow ==
  TPMSResButtAllow : Inport
  Data Type Conversion : DataTypeConversion  OutDataTypeStr=uint8  RndMeth=Round
  CAN2_TPMS_Res_Butt_Allow : Outport
  wires:
  Data Type Conversion/1 -> CAN2_TPMS_Res_Butt_Allow/1
  TPMSResButtAllow/1 -> Data Type Conversion/1

== system halout/HAL_OUT/CAN2/FD_TPMS1_0x435/TPMSWarnIndi ==
  TPMSWarnIndi : Inport
  Data Type Conversion : DataTypeConversion  OutDataTypeStr=uint8  RndMeth=Round
  CAN2_TPMSWarnIndi : Outport
  wires:
  Data Type Conversion/1 -> CAN2_TPMSWarnIndi/1
  TPMSWarnIndi/1 -> Data Type Conversion/1

== system halout/HAL_OUT/CAN2/FD_TPMS2_0x436/ID1ALTU ==
  ID1ALTU : Inport
  Data Type Conversion : DataTypeConversion  OutDataTypeStr=uint32  RndMeth=Round
  CAN2_ID1_ALTU : Outport
  wires:
  Data Type Conversion/1 -> CAN2_ID1_ALTU/1
  ID1ALTU/1 -> Data Type Conversion/1

== system halout/HAL_OUT/CAN2/FD_TPMS2_0x436/ID1LocALTU ==
  ID1LocALTU : Inport
  Data Type Conversion : DataTypeConversion  OutDataTypeStr=uint8  RndMeth=Round
  CAN2_ID1_Loc_ALTU : Outport
  wires:
  Data Type Conversion/1 -> CAN2_ID1_Loc_ALTU/1
  ID1LocALTU/1 -> Data Type Conversion/1

== system halout/HAL_OUT/CAN2/FD_TPMS2_0x436/ID1messageALTU ==
  ID1messageALTU : Inport
  Data Type Conversion : DataTypeConversion  OutDataTypeStr=uint8  RndMeth=Round
  CAN2_ID1_message_ALTU : Outport
  wires:
  Data Type Conversion/1 -> CAN2_ID1_message_ALTU/1
  ID1messageALTU/1 -> Data Type Conversion/1

== system halout/HAL_OUT/CAN2/FD_TPMS2_0x436/ID2ALTU ==
  ID2ALTU : Inport
  Data Type Conversion : DataTypeConversion  OutDataTypeStr=uint32  RndMeth=Round
  CAN2_ID2_ALTU : Outport
  wires:
  Data Type Conversion/1 -> CAN2_ID2_ALTU/1
  ID2ALTU/1 -> Data Type Conversion/1

== system halout/HAL_OUT/CAN2/FD_TPMS2_0x436/ID2LocALTU ==
  ID2LocALTU : Inport
  Data Type Conversion : DataTypeConversion  OutDataTypeStr=uint8  RndMeth=Round
  CAN2_ID2_Loc_ALTU : Outport
  wires:
  Data Type Conversion/1 -> CAN2_ID2_Loc_ALTU/1
  ID2LocALTU/1 -> Data Type Conversion/1

== system halout/HAL_OUT/CAN2/FD_TPMS2_0x436/ID2messageALTU ==
  ID2messageALTU : Inport
  Data Type Conversion : DataTypeConversion  OutDataTypeStr=uint8  RndMeth=Round
  CAN2_ID2_message_ALTU : Outport
  wires:
  Data Type Conversion/1 -> CAN2_ID2_message_ALTU/1
  ID2messageALTU/1 -> Data Type Conversion/1

== system halout/HAL_OUT/CAN2/FD_TPMS2_0x436/ID3ALTU ==
  ID3ALTU : Inport
  Data Type Conversion : DataTypeConversion  OutDataTypeStr=uint32  RndMeth=Round
  CAN2_ID3_ALTU : Outport
  wires:
  Data Type Conversion/1 -> CAN2_ID3_ALTU/1
  ID3ALTU/1 -> Data Type Conversion/1

== system halout/HAL_OUT/CAN2/FD_TPMS2_0x436/ID3LocALTU ==
  ID3LocALTU : Inport
  Data Type Conversion : DataTypeConversion  OutDataTypeStr=uint8  RndMeth=Round
  CAN2_ID3_Loc_ALTU : Outport
  wires:
  Data Type Conversion/1 -> CAN2_ID3_Loc_ALTU/1
  ID3LocALTU/1 -> Data Type Conversion/1

== system halout/HAL_OUT/CAN2/FD_TPMS2_0x436/ID3messageALTU ==
  ID3messageALTU : Inport
  Data Type Conversion : DataTypeConversion  OutDataTypeStr=uint8  RndMeth=Round
  CAN2_ID3_message_ALTU : Outport
  wires:
  Data Type Conversion/1 -> CAN2_ID3_message_ALTU/1
  ID3messageALTU/1 -> Data Type Conversion/1

== system halout/HAL_OUT/CAN2/FD_TPMS2_0x436/ID4ALTU ==
  ID4ALTU : Inport
  Data Type Conversion : DataTypeConversion  OutDataTypeStr=uint32  RndMeth=Round
  CAN2_ID4_ALTU : Outport
  wires:
  Data Type Conversion/1 -> CAN2_ID4_ALTU/1
  ID4ALTU/1 -> Data Type Conversion/1

== system halout/HAL_OUT/CAN2/FD_TPMS2_0x436/ID4LocALTU ==
  ID4LocALTU : Inport
  Data Type Conversion : DataTypeConversion  OutDataTypeStr=uint8  RndMeth=Round
  CAN2_ID4_Loc_ALTU : Outport
  wires:
  Data Type Conversion/1 -> CAN2_ID4_Loc_ALTU/1
  ID4LocALTU/1 -> Data Type Conversion/1

== system halout/HAL_OUT/CAN2/FD_TPMS2_0x436/ID4messageALTU ==
  ID4messageALTU : Inport
  Data Type Conversion : DataTypeConversion  OutDataTypeStr=uint8  RndMeth=Round
  CAN2_ID4_message_ALTU : Outport
  wires:
  Data Type Conversion/1 -> CAN2_ID4_message_ALTU/1
  ID4messageALTU/1 -> Data Type Conversion/1

== system halout/HAL_OUT/CAN2/FD_TPMS2_0x436/IDinALTU ==
  IDinALTU : Inport
  Data Type Conversion : DataTypeConversion  OutDataTypeStr=uint32  RndMeth=Round
  CAN2_IDin_ALTU : Outport
  wires:
  Data Type Conversion/1 -> CAN2_IDin_ALTU/1
  IDinALTU/1 -> Data Type Conversion/1

== system halout/HAL_OUT/CAN2/FD_TPMS2_0x436/RFFATALTU ==
  RFFATALTU : Inport
  Data Type Conversion : DataTypeConversion  OutDataTypeStr=uint8  RndMeth=Round
  CAN2_RF_FAT_ALTU : Outport
  wires:
  Data Type Conversion/1 -> CAN2_RF_FAT_ALTU/1
  RFFATALTU/1 -> Data Type Conversion/1

== system halout/HAL_OUT/CAN2/FD_TPMS2_0x436/S1WheelDebugALTU ==
  S1WheelDebugALTU : Inport
  Data Type Conversion : DataTypeConversion  OutDataTypeStr=uint8  RndMeth=Round
  convert_out : FVT_lib/hal/convert_out  gain=0.5  offset=0
  CAN2_S1WheelDebug_ALTU : Outport
  wires:
  Data Type Conversion/1 -> CAN2_S1WheelDebug_ALTU/1
  convert_out/1 -> Data Type Conversion/1
  S1WheelDebugALTU/1 -> convert_out/1

== system halout/HAL_OUT/CAN2/FD_TPMS2_0x436/S2WheelDebugALTU ==
  S2WheelDebugALTU : Inport
  Data Type Conversion : DataTypeConversion  OutDataTypeStr=uint8  RndMeth=Round
  convert_out : FVT_lib/hal/convert_out  gain=0.5  offset=0
  CAN2_S2WheelDebug_ALTU : Outport
  wires:
  Data Type Conversion/1 -> CAN2_S2WheelDebug_ALTU/1
  convert_out/1 -> Data Type Conversion/1
  S2WheelDebugALTU/1 -> convert_out/1

== system halout/HAL_OUT/CAN2/FD_TPMS2_0x436/S3WheelDebugALTU ==
  S3WheelDebugALTU : Inport
  Data Type Conversion : DataTypeConversion  OutDataTypeStr=uint8  RndMeth=Round
  convert_out : FVT_lib/hal/convert_out  gain=0.5  offset=0
  CAN2_S3WheelDebug_ALTU : Outport
  wires:
  Data Type Conversion/1 -> CAN2_S3WheelDebug_ALTU/1
  convert_out/1 -> Data Type Conversion/1
  S3WheelDebugALTU/1 -> convert_out/1

== system halout/HAL_OUT/CAN2/FD_TPMS2_0x436/S4WheelDebugALTU ==
  S4WheelDebugALTU : Inport
  Data Type Conversion : DataTypeConversion  OutDataTypeStr=uint8  RndMeth=Round
  convert_out : FVT_lib/hal/convert_out  gain=0.5  offset=0
  CAN2_S4WheelDebug_ALTU : Outport
  wires:
  Data Type Conversion/1 -> CAN2_S4WheelDebug_ALTU/1
  convert_out/1 -> Data Type Conversion/1
  S4WheelDebugALTU/1 -> convert_out/1

== system halout/HAL_OUT/CAN2/FD_V2L1_0x374/ReqOBCV2LEna ==
  ReqOBCV2LEna : Inport
  Data Type Conversion : DataTypeConversion  OutDataTypeStr=uint8  RndMeth=Round
  CAN2_Req_OBCV2LEna : Outport
  wires:
  Data Type Conversion/1 -> CAN2_Req_OBCV2LEna/1
  ReqOBCV2LEna/1 -> Data Type Conversion/1

== system halout/HAL_OUT/CAN2/FD_V2L1_0x374/ReqV2LIVIPopup ==
  ReqV2LIVIPopup : Inport
  Data Type Conversion : DataTypeConversion  OutDataTypeStr=uint8  RndMeth=Round
  CAN2_Req_V2L_IVI_Popup : Outport
  wires:
  Data Type Conversion/1 -> CAN2_Req_V2L_IVI_Popup/1
  ReqV2LIVIPopup/1 -> Data Type Conversion/1

== system halout/HAL_OUT/CAN2/FD_V2L1_0x374/ReqV2LSwOn ==
  ReqV2LSwOn : Inport
  Data Type Conversion : DataTypeConversion  OutDataTypeStr=uint8  RndMeth=Round
  CAN2_Req_V2LSwOn : Outport
  wires:
  Data Type Conversion/1 -> CAN2_Req_V2LSwOn/1
  ReqV2LSwOn/1 -> Data Type Conversion/1

== system halout/HAL_OUT/CAN2/FD_VCU0_0x1F0/EVCCAplusPwrUpReq ==
  EVCCAplusPwrUpReq : Inport
  Data Type Conversion : DataTypeConversion  OutDataTypeStr=uint8  RndMeth=Round
  CAN2_EVCCAplusPwrUpReq : Outport
  wires:
  Data Type Conversion/1 -> CAN2_EVCCAplusPwrUpReq/1
  EVCCAplusPwrUpReq/1 -> Data Type Conversion/1

== system halout/HAL_OUT/CAN2/FD_VCU0_0x1F0/FDADC12VDetAvg ==
  FDADC12VDetAvg : Inport
  Data Type Conversion : DataTypeConversion  OutDataTypeStr=uint8  RndMeth=Round
  convert_out : FVT_lib/hal/convert_out  gain=0.1  offset=0
  CAN2_FDADC12VDetAvg : Outport
  wires:
  Data Type Conversion/1 -> CAN2_FDADC12VDetAvg/1
  convert_out/1 -> Data Type Conversion/1
  FDADC12VDetAvg/1 -> convert_out/1

== system halout/HAL_OUT/CAN2/FD_VCU0_0x1F0/FrTqSource ==
  FrTqSource : Inport
  Data Type Conversion : DataTypeConversion  OutDataTypeStr=uint8  RndMeth=Round
  CAN2_Fr_TqSource : Outport
  wires:
  Data Type Conversion/1 -> CAN2_Fr_TqSource/1
  FrTqSource/1 -> Data Type Conversion/1

== system halout/HAL_OUT/CAN2/FD_VCU0_0x1F0/HVRlyOpFail ==
  HVRlyOpFail : Inport
  Data Type Conversion : DataTypeConversion  OutDataTypeStr=uint8  RndMeth=Round
  CAN2_HVRlyOpFail : Outport
  wires:
  Data Type Conversion/1 -> CAN2_HVRlyOpFail/1
  HVRlyOpFail/1 -> Data Type Conversion/1

== system halout/HAL_OUT/CAN2/FD_VCU0_0x1F0/HVTHCMSysAvail ==
  HVTHCMSysAvail : Inport
  Data Type Conversion : DataTypeConversion  OutDataTypeStr=uint8  RndMeth=Round
  CAN2_HVTHCMSysAvail : Outport
  wires:
  Data Type Conversion/1 -> CAN2_HVTHCMSysAvail/1
  HVTHCMSysAvail/1 -> Data Type Conversion/1

== system halout/HAL_OUT/CAN2/FD_VCU0_0x1F0/LVBattChrgtimeAct ==
  LVBattChrgtimeAct : Inport
  Data Type Conversion : DataTypeConversion  OutDataTypeStr=uint16  RndMeth=Round
  CAN2_LVBattChrgtimeAct : Outport
  wires:
  Data Type Conversion/1 -> CAN2_LVBattChrgtimeAct/1
  LVBattChrgtimeAct/1 -> Data Type Conversion/1

== system halout/HAL_OUT/CAN2/FD_VCU0_0x1F0/LVBattVoltSta ==
  LVBattVoltSta : Inport
  Data Type Conversion : DataTypeConversion  OutDataTypeStr=uint8  RndMeth=Round
  CAN2_LVBattVoltSta : Outport
  wires:
  Data Type Conversion/1 -> CAN2_LVBattVoltSta/1
  LVBattVoltSta/1 -> Data Type Conversion/1

== system halout/HAL_OUT/CAN2/FD_VCU0_0x1F0/LVChrgHoldTAct ==
  LVChrgHoldTAct : Inport
  Data Type Conversion : DataTypeConversion  OutDataTypeStr=uint16  RndMeth=Round
  CAN2_LVChrgHoldTAct : Outport
  wires:
  Data Type Conversion/1 -> CAN2_LVChrgHoldTAct/1
  LVChrgHoldTAct/1 -> Data Type Conversion/1

== system halout/HAL_OUT/CAN2/FD_VCU0_0x1F0/LVSilentChrgLv ==
  LVSilentChrgLv : Inport
  Data Type Conversion : DataTypeConversion  OutDataTypeStr=uint8  RndMeth=Round
  CAN2_LVSilentChrgLv : Outport
  wires:
  Data Type Conversion/1 -> CAN2_LVSilentChrgLv/1
  LVSilentChrgLv/1 -> Data Type Conversion/1

== system halout/HAL_OUT/CAN2/FD_VCU0_0x1F0/LVSilentChrgReq ==
  LVSilentChrgReq : Inport
  Data Type Conversion : DataTypeConversion  OutDataTypeStr=uint8  RndMeth=Round
  CAN2_LVSilentChrgReq : Outport
  wires:
  Data Type Conversion/1 -> CAN2_LVSilentChrgReq/1
  LVSilentChrgReq/1 -> Data Type Conversion/1

== system halout/HAL_OUT/CAN2/FD_VCU0_0x1F0/LVSilentChrgSta ==
  LVSilentChrgSta : Inport
  Data Type Conversion : DataTypeConversion  OutDataTypeStr=uint8  RndMeth=Round
  CAN2_LVSilentChrgSta : Outport
  wires:
  Data Type Conversion/1 -> CAN2_LVSilentChrgSta/1
  LVSilentChrgSta/1 -> Data Type Conversion/1

== system halout/HAL_OUT/CAN2/FD_VCU0_0x1F0/MCUActDisFail ==
  MCUActDisFail : Inport
  Data Type Conversion : DataTypeConversion  OutDataTypeStr=uint8  RndMeth=Round
  CAN2_MCUActDisFail : Outport
  wires:
  Data Type Conversion/1 -> CAN2_MCUActDisFail/1
  MCUActDisFail/1 -> Data Type Conversion/1

== system halout/HAL_OUT/CAN2/FD_VCU0_0x1F0/PMMAllowECUSleep ==
  PMMAllowECUSleep : Inport
  Data Type Conversion : DataTypeConversion  OutDataTypeStr=uint8  RndMeth=Round
  CAN2_PMMAllowECUSleep : Outport
  wires:
  Data Type Conversion/1 -> CAN2_PMMAllowECUSleep/1
  PMMAllowECUSleep/1 -> Data Type Conversion/1

== system halout/HAL_OUT/CAN2/FD_VCU0_0x1F0/PowerDownFault ==
  PowerDownFault : Inport
  Data Type Conversion : DataTypeConversion  OutDataTypeStr=uint8  RndMeth=Round
  CAN2_PowerDownFault : Outport
  wires:
  Data Type Conversion/1 -> CAN2_PowerDownFault/1
  PowerDownFault/1 -> Data Type Conversion/1

== system halout/HAL_OUT/CAN2/FD_VCU0_0x1F0/PowerDownState ==
  PowerDownState : Inport
  Data Type Conversion : DataTypeConversion  OutDataTypeStr=uint8  RndMeth=Round
  CAN2_PowerDownState : Outport
  wires:
  Data Type Conversion/1 -> CAN2_PowerDownState/1
  PowerDownState/1 -> Data Type Conversion/1

== system halout/HAL_OUT/CAN2/FD_VCU0_0x1F0/PowerUpFault ==
  PowerUpFault : Inport
  Data Type Conversion : DataTypeConversion  OutDataTypeStr=uint8  RndMeth=Round
  CAN2_PowerUpFault : Outport
  wires:
  Data Type Conversion/1 -> CAN2_PowerUpFault/1
  PowerUpFault/1 -> Data Type Conversion/1

== system halout/HAL_OUT/CAN2/FD_VCU0_0x1F0/PowerUpState ==
  PowerUpState : Inport
  Data Type Conversion : DataTypeConversion  OutDataTypeStr=uint8  RndMeth=Round
  CAN2_PowerUpState : Outport
  wires:
  Data Type Conversion/1 -> CAN2_PowerUpState/1
  PowerUpState/1 -> Data Type Conversion/1

== system halout/HAL_OUT/CAN2/FD_VCU0_0x1F0/PwrDownReq ==
  PwrDownReq : Inport
  Data Type Conversion : DataTypeConversion  OutDataTypeStr=uint8  RndMeth=Round
  CAN2_PwrDownReq : Outport
  wires:
  Data Type Conversion/1 -> CAN2_PwrDownReq/1
  PwrDownReq/1 -> Data Type Conversion/1

== system halout/HAL_OUT/CAN2/FD_VCU0_0x1F0/PwrStaConstraint ==
  PwrStaConstraint : Inport
  Data Type Conversion : DataTypeConversion  OutDataTypeStr=uint8  RndMeth=Round
  CAN2_PwrStaConstraint : Outport
  wires:
  Data Type Conversion/1 -> CAN2_PwrStaConstraint/1
  PwrStaConstraint/1 -> Data Type Conversion/1

== system halout/HAL_OUT/CAN2/FD_VCU0_0x1F0/PwrStaONTOIVIPopReq ==
  PwrStaONTOIVIPopReq : Inport
  Data Type Conversion : DataTypeConversion  OutDataTypeStr=uint8  RndMeth=Round
  CAN2_PwrStaONTOIVIPopReq : Outport
  wires:
  Data Type Conversion/1 -> CAN2_PwrStaONTOIVIPopReq/1
  PwrStaONTOIVIPopReq/1 -> Data Type Conversion/1

== system halout/HAL_OUT/CAN2/FD_VCU0_0x1F0/PwrStaONTOIVIPopT ==
  PwrStaONTOIVIPopT : Inport
  Data Type Conversion : DataTypeConversion  OutDataTypeStr=uint16  RndMeth=Round
  CAN2_PwrStaONTOIVIPopT : Outport
  wires:
  Data Type Conversion/1 -> CAN2_PwrStaONTOIVIPopT/1
  PwrStaONTOIVIPopT/1 -> Data Type Conversion/1

== system halout/HAL_OUT/CAN2/FD_VCU0_0x1F0/PwrStaSelect ==
  PwrStaSelect : Inport
  Data Type Conversion : DataTypeConversion  OutDataTypeStr=uint8  RndMeth=Round
  CAN2_PwrStaSelect : Outport
  wires:
  Data Type Conversion/1 -> CAN2_PwrStaSelect/1
  PwrStaSelect/1 -> Data Type Conversion/1

== system halout/HAL_OUT/CAN2/FD_VCU0_0x1F0/PwrStaTOSta ==
  PwrStaTOSta : Inport
  Data Type Conversion : DataTypeConversion  OutDataTypeStr=uint8  RndMeth=Round
  CAN2_PwrStaTOSta : Outport
  wires:
  Data Type Conversion/1 -> CAN2_PwrStaTOSta/1
  PwrStaTOSta/1 -> Data Type Conversion/1

== system halout/HAL_OUT/CAN2/FD_VCU0_0x1F0/PwrUpReq ==
  PwrUpReq : Inport
  Data Type Conversion : DataTypeConversion  OutDataTypeStr=uint8  RndMeth=Round
  CAN2_PwrUpReq : Outport
  wires:
  Data Type Conversion/1 -> CAN2_PwrUpReq/1
  PwrUpReq/1 -> Data Type Conversion/1

== system halout/HAL_OUT/CAN2/FD_VCU0_0x1F0/RrTqSource ==
  RrTqSource : Inport
  Data Type Conversion : DataTypeConversion  OutDataTypeStr=uint8  RndMeth=Round
  CAN2_Rr_TqSource : Outport
  wires:
  Data Type Conversion/1 -> CAN2_Rr_TqSource/1
  RrTqSource/1 -> Data Type Conversion/1

== system halout/HAL_OUT/CAN2/FD_VCU0_0x1F0/SchedChgTOSta ==
  SchedChgTOSta : Inport
  Data Type Conversion : DataTypeConversion  OutDataTypeStr=uint8  RndMeth=Round
  CAN2_SchedChgTOSta : Outport
  wires:
  Data Type Conversion/1 -> CAN2_SchedChgTOSta/1
  SchedChgTOSta/1 -> Data Type Conversion/1

== system halout/HAL_OUT/CAN2/FD_VCU0_0x1F0/SilentChkAllowSleep ==
  SilentChkAllowSleep : Inport
  Data Type Conversion : DataTypeConversion  OutDataTypeStr=uint8  RndMeth=Round
  CAN2_SilentChkAllowSleep : Outport
  wires:
  Data Type Conversion/1 -> CAN2_SilentChkAllowSleep/1
  SilentChkAllowSleep/1 -> Data Type Conversion/1
